simulink model "PID_Controller"  (R2020a)
settings: Solver=ode45  StartTime=0.0  StopTime=10  RelTol=1e-6  AbsTol=1e-6
values from neighbouring files (symbols this model uses):
  f = 1e-1    (= 0.1)    [Initialisation_PID.m]
  J = 1e-2    (= 0.01)    [Initialisation_PID.m]
  k = 0.05    [Initialisation_PID.m]
  L = 1e-1    (= 0.1)    [Initialisation_PID.m]
  R = 50    [Initialisation_PID.m]    (also in Initialization_Kalman.m = [Sensor_noise(1)^2 0; 0 Sensor_noise(2)^2]; Kalman_Matlab.m = [Sensor_noise(1)^2 0; 0 Sensor_noise(2)^2])
libraries: simulink x1
settings Model: Creator=Alexis  LastModifiedBy=Welcome
settings SolverCC: AutoScaleAbsTol=off  ShapePreserveControl=EnableAll  ZeroCrossAlgorithm=Adaptive
settings DataIOCC: ReturnWorkspaceOutputs=off
settings DebuggingCC: ArithmeticOperatorsInVariantConditions=warning
settings SFSimCC: SimUseLocalCustomCode=off  CustomCodeUndefinedFunction=UseInterfaceOnly
settings RTWCC: RTWUseLocalCustomCode=off
settings CodeAppCC: StateflowObjectComments=on

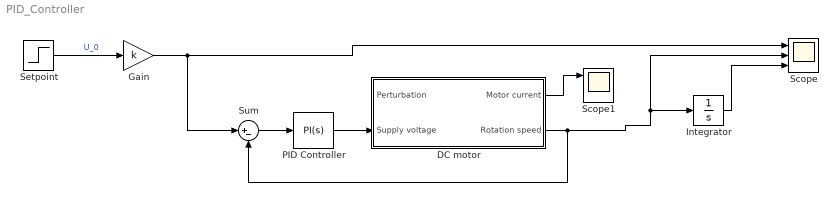
== system PID_Controller ==
  DC motor : Subsystem
  Gain : Gain  Gain=k
  Integrator : Integrator
  PID Controller : simulink/Continuous/PID Controller  Controller=PI  Form=Parallel  TimeDomain=Continuous-time  UseExternalTs=off  SampleTime=-1  IntegratorMethod=Forward Euler  FilterMethod=Forward Euler  ControllerParametersSource=internal  P=21.8728908491505  I=5409.87686032159  D=1.5  UseFilter=on  N=5  TunerSelectOption=Transfer Function Based (PID Tuner App)  InitialConditionSource=internal  InitialConditionForIntegrator=0  InitialConditionForFilter=0  DifferentiatorICPrevScaledInput=0  ExternalReset=none  TrackingMode=off  Kt=1  LimitOutput=off  UpperSaturationLimit=inf  LowerSaturationLimit=-inf  LinearizeAsGain=on  AntiWindupMode=none  Kb=1  POutMin=[]  POutMax=[]  IOutMin=[]  IOutMax=[]  DOutMin=[]  DOutMax=[]  NOutMin=[]  NOutMax=[]  SumOutMin=[]  SumOutMax=[]  SaturationOutMin=[]  SaturationOutMax=[]  PParamMin=[]  PParamMax=[]  IParamMin=[]  IParamMax=[]  DParamMin=[]  DParamMax=[]  NParamMin=[]  NParamMax=[]  KbParamMin=[]  KbParamMax=[]  KtParamMin=[]  KtParamMax=[]  KbOutMin=[]  KbOutMax=[]  KtOutMin=[]  KtOutMax=[]  IntegratorOutMin=[]  IntegratorOutMax=[]  FilterOutMin=[]  FilterOutMax=[]  SumI1OutMin=[]  SumI1OutMax=[]  SumI2OutMin=[]  SumI2OutMax=[]  SumI3OutMin=[]  SumI3OutMax=[]  SumI4OutMin=[]  SumI4OutMax=[]  SumDOutMin=[]  SumDOutMax=[]  DifferentiatorOutMin=[]  DifferentiatorOutMax=[]  FilterDiffOutCoefMin=[]  FilterDiffOutCoefMax=[]  ReciprocalOutMin=[]  ReciprocalOutMax=[]  SumDenOutMin=[]  SumDenOutMax=[]  SumNumOutMin=[]  SumNumOutMax=[]  DivideOutMin=[]  DivideOutMax=[]  UdiffTsProdOutMin=[]  UdiffTsProdOutMax=[]  NTsProdOutMin=[]  NTsProdOutMax=[]  UintegralTsProdOutMin=[]  UintegralTsProdOutMax=[]  UngainTsProdOutMin=[]  UngainTsProdOutMax=[]  IntegratorContinuousStateAttributes=''  IntegratorStateMustResolveToSignalObject=off  IntegratorRTWStateStorageClass=Auto  FilterContinuousStateAttributes=''  FilterStateMustResolveToSignalObject=off  FilterRTWStateStorageClass=Auto  ParallelPVariant=InternalParameters  IdealPVariant=Disabled  IVariant=InternalParameters  DVariant=Disabled  IntegratorVariant=Continuous  SatVariant=Disabled  AWVariant=Passthrough  PCopyVariant=Disabled  TRVariant=Disabled  FdbkBlocksVariant=Forward  IdealPFdbkVariant=Disabled  SatFdbkVariant=Disabled  DerivativeFilterVariant=Disabled  NVariant=Disabled  NCopyVariant=Disabled_SignalSpec  FilterICVariant=Disabled  IntegratorICVariant=InternalICs  ExternalResetVariant=Disabled  TRSumVariant=Passthrough  SumFdbkVariant=Disabled  SumVariant=Sum_PI  TsampFilterVariant=InternalTs  TsampNgainVariant=Passthrough  TsampIntegralVariant=Passthrough
  Scope : Scope  NumInputPorts=3
  Scope1 : Scope  NumInputPorts=3
  Setpoint : Step  After=20  SampleTime=0
  Sum : Sum  Inputs=|+-
  wires:
  Integrator/1 -> Scope/3
  DC motor/1(Motor current) -> Scope1/1
  DC motor/2(Rotation speed) -> Scope/2, Integrator/1, Sum/2
  Sum/1 -> PID Controller/1
  Setpoint/1 -> Gain/1  "U_0"
  Gain/1 -> Sum/1, Scope/1
  PID Controller/1 -> DC motor/2(Supply voltage)

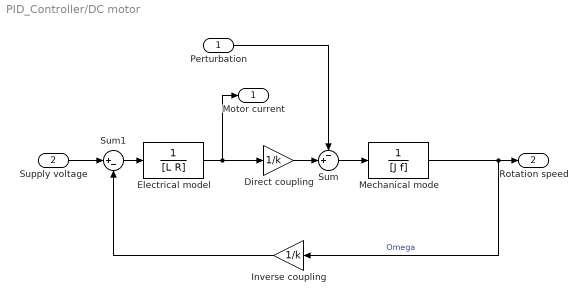
== system PID_Controller/DC motor ==
  Perturbation : Inport
  Supply voltage : Inport  Port=2
  Direct coupling : Gain  Gain=1/k
  Electrical model : TransferFcn  Denominator=[L R]
  Inverse coupling : Gain  Gain=1/k
  Mechanical mode : TransferFcn  Denominator=[J f]
  Sum : Sum  Inputs=-+|
  Sum1 : Sum  Inputs=|+-
  Motor current : Outport
  Rotation speed : Outport  Port=2
  wires:
  Direct coupling/1 -> Sum/2
  Sum/1 -> Mechanical mode/1
  Mechanical mode/1 -> Rotation speed/1, Inverse coupling/1  "Omega"
  Sum1/1 -> Electrical model/1
  Inverse coupling/1 -> Sum1/2
  Perturbation/1 -> Sum/1
  Supply voltage/1 -> Sum1/1
  Electrical model/1 -> Direct coupling/1, Motor current/1
